simulink library "flight_dynamics_models"  (R2018b)
settings: Solver=VariableStepAuto  StartTime=0.0  StopTime=10.0  RelTol=1e-3
undefined symbols (not defined in the file or in its folder): aircraft, ic
libraries: vlm_wing_lib x12, flight_parameters_lib x4, axes_transformation_lib x4, fuselage_lib x4, wing_downwash_lib x4, se2a_actuators_lib x4, $bdroot x2, flexibleBody_lib x2, rigidBody_lib x2
(part 2 of 2)

== matlab function flight_dynamics_models/Rigid aircraft with steady aerodynamics/Aerodynamics/MATLAB Function4 ==
  data: V_ext_local input; V_ext_local output; w_downwash input
function V_ext_local  = fcn(V_ext_local ,w_downwash)

V_ext_local(3,:) = V_ext_local(3,:) + w_downwash;

end
